simulink model "mdl_VD_dt7dofModel_PPC"  (R2019b)
settings: Solver=ode4  StartTime=0.0  StopTime=50  FixedStep=0.01  RelTol=1e-4  EnableMultiTasking=on
undefined symbols (not defined in the file or in its folder): controller, initial, inputTrajectory, mdlParam, road_properties, vdParam, vehicle
libraries: simulink x9
(part 1 of 2)
settings Model: Creator=cbeal  LastModifiedBy=prasa
settings SolverCC: ZeroCrossAlgorithm=Adaptive
settings DataIOCC: SaveFormat=Array  SaveTime=off  ReturnWorkspaceOutputs=off
settings OptimizationCC: ExpressionDepthLimit=2147483647  LifeSpan=inf
settings DebuggingCC: ReadBeforeWriteMsg=DisableAll  WriteAfterWriteMsg=DisableAll  WriteAfterReadMsg=DisableAll  UnderspecifiedInitializationDetection=Classic  MergeDetectMultiDrivingBlocksExec=none  SolverPrmCheckMsg=warning  MultiTaskDSMMsg=none  FcnCallInpInsideContextMsg=warning  StateNameClashWarn=warning  SFUnexpectedBacktrackingDiag=warning  SFNoUnconditionalDefaultTransitionDiag=warning  SFExecutionAtInitializationDiag=none  ArithmeticOperatorsInVariantConditions=warning
settings HardwareCC: ProdBitPerPointer=32  ProdBitPerSizeT=32  ProdBitPerPtrDiffT=32  ProdLargestAtomicFloat=None  ProdIntDivRoundTo=Undefined  ProdEndianess=Unspecified  ProdWordSize=32  ProdHWDeviceType=32-bit Generic
settings ModelReferenceCC: UpdateModelReferenceTargets=IfOutOfDate  PropagateSignalLabelsOutOfModel=off
settings SFSimCC: SFSimEcho=off  SimUseLocalCustomCode=off  CustomCodeUndefinedFunction=UseInterfaceOnly
settings RTWCC: RTWUseLocalCustomCode=off
settings CodeAppCC: StateflowObjectComments=on
settings GRTTargetCC: TargetLangStandard=C89/C90 (ANSI)
settings ConfigComp: CovMetricSettings=dw  CovHtmlReporting=on  CovSaveCumulativeToWorkspaceVar=on  CovSaveSingleToWorkspaceVar=on  CovExternalEMLEnable=off

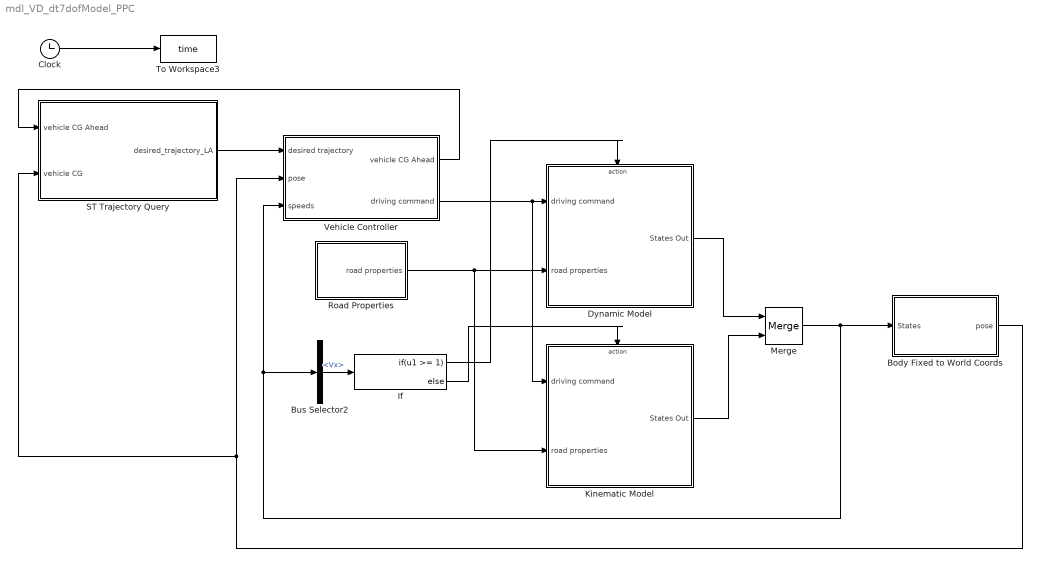
== system mdl_VD_dt7dofModel_PPC ==
  Body Fixed to World Coords : Subsystem
      mask Display: image('$imagefile'); % Use "Edit Image" on toolstrip to change.
  Bus Selector2 : BusSelector  OutputSignals=speeds.Vx
  Clock : Clock
  Dynamic Model : Subsystem
  If : If  IfExpression=u1 >= 1
  Kinematic Model : Subsystem
  Merge : Merge
  Road Properties : Subsystem
  ST Trajectory Query : Subsystem
  To Workspace3 : ToWorkspace  VariableName=time  SampleTime=-1
  Vehicle Controller : Subsystem
  wires:
  Clock/1 -> To Workspace3/1
  Vehicle Controller/2(driving command) -> Kinematic Model/1(driving command), Dynamic Model/1(driving command)
  Road Properties/1(road properties) -> Kinematic Model/2(road properties), Dynamic Model/2(road properties)
  Merge/1 -> Body Fixed to World Coords/1(States), Bus Selector2/1, Vehicle Controller/3(speeds)
  Body Fixed to World Coords/1(pose) -> Vehicle Controller/2(pose), ST Trajectory Query/2(vehicle CG)
  ST Trajectory Query/1(desired_trajectory_LA) -> Vehicle Controller/1(desired trajectory)
  Vehicle Controller/1(vehicle CG Ahead) -> ST Trajectory Query/1(vehicle CG Ahead)
  If/1 -> Dynamic Model/Action
  If/2 -> Kinematic Model/Action
  Bus Selector2/1 -> If/1  "<Vx>"
  Kinematic Model/1(States Out) -> Merge/2
  Dynamic Model/1(States Out) -> Merge/1

== system mdl_VD_dt7dofModel_PPC/Body Fixed to World Coords ==
  States : Inport
  Bus Creator1 : BusCreator  Inputs=3
  Bus Selector4 : BusSelector  OutputSignals=speeds.Vx,speeds.Vy,speeds.r
  Integrator_East : Integrator  InitialCondition=initial.east
  Integrator_North : Integrator  InitialCondition=initial.north
  Integrator_Psi : Integrator  InitialCondition=initial.heading
  Product{4..7} (4 alike) : Product  SaturateOnIntegerOverflow=on  OutDataTypeStr=Inherit: Same as first input
  Sum : Sum  Inputs=+-  SaturateOnIntegerOverflow=on
  Sum1 : Sum  SaturateOnIntegerOverflow=on
  Trigonometric Function2 : Trigonometry
  Trigonometric Function3 : Trigonometry  Operator=cos
  pose : Outport
  wires:
  Bus Creator1/1 -> pose/1
  Product4/1 -> Sum1/1
  Product6/1 -> Sum/2
  Product7/1 -> Sum1/2
  Trigonometric Function2/1 -> Product4/2, Product6/2
  Integrator_Psi/1 -> Bus Creator1/3, Trigonometric Function3/1, Trigonometric Function2/1  "PSI"
  Sum1/1 -> Integrator_North/1
  Sum/1 -> Integrator_East/1
  Trigonometric Function3/1 -> Product5/2, Product7/2
  Integrator_East/1 -> Bus Creator1/1  "East"
  Product5/1 -> Sum/1
  Integrator_North/1 -> Bus Creator1/2  "North"
  Bus Selector4/1 -> Product4/1, Product5/1  "<Vx>"
  Bus Selector4/3 -> Integrator_Psi/1  "<r>"
  Bus Selector4/2 -> Product7/1, Product6/1  "<Vy>"
  States/1 -> Bus Selector4/1

== system mdl_VD_dt7dofModel_PPC/Dynamic Model ==
  driving command : Inport
  road properties : Inport  Port=2
  Action Port : ActionPort  ActionPortLabel=if(u1 >= 1)
  Brush Model : Subsystem
  Normal Force : Subsystem
      mask Display: image('$imagefile'); % Use "Edit Image" on toolstrip to change.
  Slips : Subsystem
      mask Display: image('$imagefile'); % Use "Edit Image" on toolstrip to change.
  Vehicle Body Newtonian Dynamics : Subsystem
      mask Display: image('$imagefile'); % Use "Edit Image" on toolstrip to change.
  States Out : Outport
  wires:
  road properties/1 -> Vehicle Body Newtonian Dynamics/3(Road Geometry), Brush Model/3(Road Friction), Normal Force/2(road properties)
  Normal Force/1(Normal Forces) -> Brush Model/2(Normal Forces)  "Normal Forces"
  Vehicle Body Newtonian Dynamics/1(States_Out) -> States Out/1, Vehicle Body Newtonian Dynamics/4(States_IN), Slips/2(Speeds), Normal Force/1(Accelerations)
  Slips/1(Slips) -> Brush Model/1(Slips)  "Slips"
  driving command/1 -> Vehicle Body Newtonian Dynamics/1(Driving Command), Slips/1(steering angle)
  Brush Model/1(Tire Forces) -> Vehicle Body Newtonian Dynamics/2(Tire Forces)

== system mdl_VD_dt7dofModel_PPC/Kinematic Model ==
  driving command : Inport
  road properties : Inport  Port=2
  Action Port : ActionPort  ActionPortLabel=else
  Constant : Constant  Value=0.015
  Normal Force : Subsystem
      mask Display: image('$imagefile'); % Use "Edit Image" on toolstrip to change.
  Product13 : Product  RndMeth=Zero
  Vehicle Body Newtonian Dynamics : Subsystem
      mask Display: image('$imagefile'); % Use "Edit Image" on toolstrip to change.
  States Out : Outport
  wires:
  road properties/1 -> Vehicle Body Newtonian Dynamics/3(Road Geometry), Normal Force/2(road properties)
  Normal Force/1(Normal Forces) -> Product13/2  "Normal Forces"
  Vehicle Body Newtonian Dynamics/1(States_Out) -> Normal Force/1(Accelerations), States Out/1
  driving command/1 -> Vehicle Body Newtonian Dynamics/1(Driving Command)
  Product13/1 -> Vehicle Body Newtonian Dynamics/2(Rolling Resistance Force)  "Resistive Forces"
  Constant/1 -> Product13/1

== system mdl_VD_dt7dofModel_PPC/Road Properties ==
  Bus Creator1 : BusCreator  Inputs=3
  Bus Creator2 : BusCreator  Inputs=2
  Constant : Constant  Value=road_properties.friction
  Constant1 : Constant  Value=road_properties.grade
  Constant19 : Constant  Value=road_properties.bank_angle
  Constant3 : Constant  Value=0
  road properties : Outport
  wires:
  Constant1/1 -> Bus Creator1/2  "grade"
  Constant19/1 -> Bus Creator1/1  "banking angle"
  Constant3/1 -> Bus Creator1/3  "Curvature"
  Constant/1 -> Bus Creator2/2  "road friction"
  Bus Creator2/1 -> road properties/1  "road properties"
  Bus Creator1/1 -> Bus Creator2/1  "road geometry"

== system mdl_VD_dt7dofModel_PPC/ST Trajectory Query ==
  vehicle CG Ahead : Inport
  vehicle CG : Inport  Port=2
  Constant1 : Constant  Value=mdlParam.max_station
  IsNegative1 : simulink/Logic and Bit Operations/Compare To Zero  relop=<  OutDataTypeStr=boolean
  IsNonNegative1 : simulink/Logic and Bit Operations/Compare To Zero  relop=>=  OutDataTypeStr=boolean
  ST Trajectory Query1 : Subsystem
  ST Trajectory Query2 : Subsystem
  Stop Simulation2 : Stop
  Stop Simulation3 : Stop
  Subtract2 : Sum  Inputs=-+
  Subtract3 : Sum  Inputs=-+
  To Workspace3 : ToWorkspace  VariableName=desired_trajectory  SampleTime=-1
  desired_trajectory_LA : Outport
  wires:
  ST Trajectory Query2/2(desired_trajectory_LA) -> To Workspace3/1, desired_trajectory_LA/1
  vehicle CG/1 -> ST Trajectory Query1/1(vehicle CG(EN))
  vehicle CG Ahead/1 -> ST Trajectory Query2/1(vehicle CG Ahead(EN))
  IsNegative1/1 -> Stop Simulation3/1
  Subtract3/1 -> IsNegative1/1
  Constant1/1 -> Subtract2/1
  IsNonNegative1/1 -> Stop Simulation2/1
  Subtract2/1 -> IsNonNegative1/1
  ST Trajectory Query2/1(vehicle station ahead) -> Subtract3/2
  ST Trajectory Query1/1(vehicle station current) -> Subtract2/2, Subtract3/1

== system mdl_VD_dt7dofModel_PPC/Vehicle Controller ==
  desired trajectory : Inport
  pose : Inport  Port=2
  speeds : Inport  Port=3
  Driver Model : Subsystem
      mask Display: image('$imagefile'); % Use "Edit Image" on toolstrip to change.
  Stabilization : Subsystem
  vehicle CG Ahead : Outport
  driving command : Outport  Port=2
  wires:
  Stabilization/1(driving command) -> driving command/1
  desired trajectory/1 -> Driver Model/1(desired trajectory)
  Driver Model/1(delta) -> Stabilization/1(delta_in)
  Driver Model/2(wheel torque) -> Stabilization/2(wheel torque_in)
  pose/1 -> Driver Model/2(pose)
  Driver Model/3(vehicle CG Ahead) -> vehicle CG Ahead/1
  speeds/1 -> Driver Model/3(speeds)

== system mdl_VD_dt7dofModel_PPC/Dynamic Model/Brush Model ==
  Slips : Inport
  Normal Forces : Inport  Port=2
  Road Friction : Inport  Port=3
  Tire Forces_Brush Model : Subsystem
      mask Display: image('$imagefile'); % Use "Edit Image" on toolstrip to change.
  Tire Forces : Outport
  wires:
  Road Friction/1 -> Tire Forces_Brush Model/3(road friction)
  Tire Forces_Brush Model/1(Tire Forces) -> Tire Forces/1  "Tire Forces"
  Normal Forces/1 -> Tire Forces_Brush Model/2(Normal Forces)
  Slips/1 -> Tire Forces_Brush Model/1(Slips)

== system mdl_VD_dt7dofModel_PPC/Dynamic Model/Normal Force ==
  Accelerations : Inport
  road properties : Inport  Port=2
  Left Front : Sum  Inputs=+--
  Left Rear : Sum  Inputs=++-
  Mux : Mux
  Normal Force Lateral Transfer : Subsystem
      mask Display: image('$imagefile'); % Use "Edit Image" on toolstrip to change.
  Normal Force Longitudinal Transfer : Subsystem
      mask Display: image('$imagefile'); % Use "Edit Image" on toolstrip to change.
  Normal Force Static : Subsystem
  Right Front : Sum  Inputs=+-+
  Right Rear : Sum  Inputs=+++
  To Workspace1 : ToWorkspace  VariableName=Fz  SampleTime=-1
  Normal Forces : Outport
  wires:
  Left Front/1 -> Mux/1
  Right Front/1 -> Mux/2
  Left Rear/1 -> Mux/3
  Right Rear/1 -> Mux/4
  Normal Force Static/4(Static RR) -> Right Rear/1
  Normal Force Static/1(Static FL) -> Left Front/1
  road properties/1 -> Normal Force Static/1(Road Geometry)
  Normal Force Longitudinal Transfer/1(Long Transfer) -> Left Front/2, Right Front/2, Left Rear/2, Right Rear/2
  Accelerations/1 -> Normal Force Lateral Transfer/1(Accelerations), Normal Force Longitudinal Transfer/1(Accelerations)
  Normal Force Lateral Transfer/2(Lateral Transfer Rear) -> Left Rear/3, Right Rear/3
  Normal Force Lateral Transfer/1(Lateral Transfer Front) -> Left Front/3, Right Front/3
  Normal Force Static/3(Static RL) -> Left Rear/1
  Normal Force Static/2(Static FR) -> Right Front/1
  Mux/1 -> To Workspace1/1, Normal Forces/1  "Normal Forces"

== system mdl_VD_dt7dofModel_PPC/Dynamic Model/Slips ==
  steering angle : Inport
  Speeds : Inport  Port=2
  Bus Creator : BusCreator  Inputs=2
  Bus Selector1 : BusSelector  OutputSignals=speeds
  Bus Selector2 : BusSelector  OutputSignals=steering angle
  Slip Angle : Subsystem
      mask Display: image('$imagefile'); % Use "Edit Image" on toolstrip to change.
  To Workspace : ToWorkspace  VariableName=alpha  SampleTime=-1
  To Workspace4 : ToWorkspace  VariableName=kappa  SampleTime=-1
  Wheel Slip Ratio : Subsystem
      mask Display: image('$imagefile'); % Use "Edit Image" on toolstrip to change.
  Slips : Outport
  wires:
  Slip Angle/1(Slip Angles) -> To Workspace/1, Bus Creator/1  "Slip Angles"
  Bus Selector2/1 -> Wheel Slip Ratio/1(delta), Slip Angle/2(delta)  "<steering angle>"
  Wheel Slip Ratio/1(Wheel Slips) -> To Workspace4/1, Bus Creator/2  "Wheel Slips"
  Bus Selector1/1 -> Slip Angle/1(Speeds), Wheel Slip Ratio/2(Speeds)  "<speeds>"
  Bus Creator/1 -> Slips/1
  Speeds/1 -> Bus Selector1/1
  steering angle/1 -> Bus Selector2/1

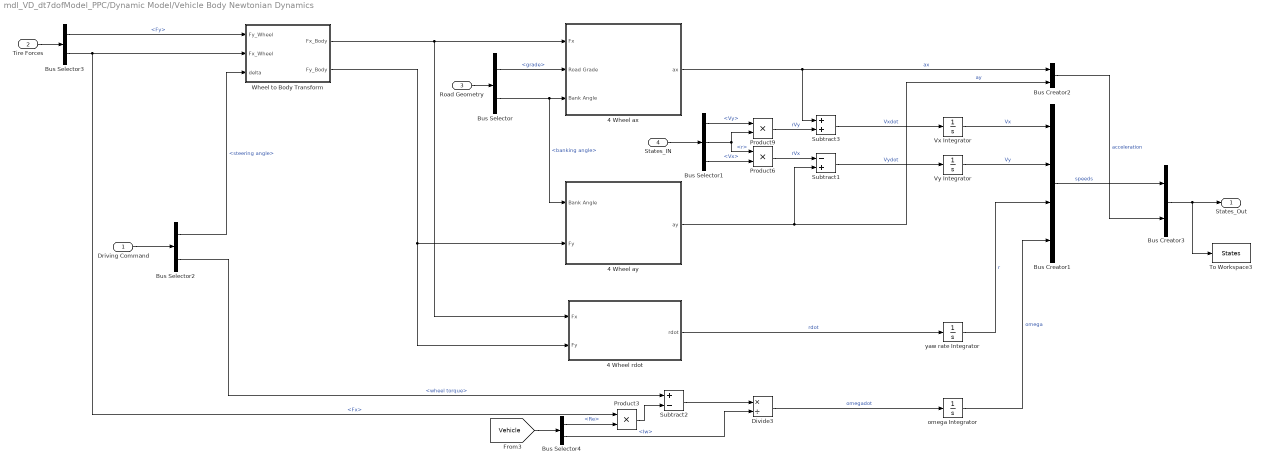
== system mdl_VD_dt7dofModel_PPC/Dynamic Model/Vehicle Body Newtonian Dynamics ==
  Driving Command : Inport
  Tire Forces : Inport  Port=2
  Road Geometry : Inport  Port=3
  States_IN : Inport  Port=4
  4 Wheel ax : Subsystem
  4 Wheel ay : Subsystem
  4 Wheel rdot : Subsystem
  Bus Creator1 : BusCreator  Inputs=4
  Bus Creator2 : BusCreator  Inputs=2
  Bus Creator3 : BusCreator  Inputs=2
  Bus Selector : BusSelector  OutputSignals=road geometry.grade,road geometry.banking angle
  Bus Selector1 : BusSelector  OutputSignals=speeds.Vy,speeds.r,speeds.Vx
  Bus Selector2 : BusSelector  OutputSignals=steering angle,wheel torque
  Bus Selector3 : BusSelector  OutputSignals=Fy,Fx
  Bus Selector4 : BusSelector  OutputSignals=Re,Iw
  Divide3 : Product  Inputs=*/
  Product3 : Product  RndMeth=Zero
  Product6 : Product  RndMeth=Zero
  Product9 : Product  RndMeth=Zero
  Subtract1 : Sum  Inputs=-+
  Subtract2 : Sum  Inputs=+-
  Subtract3 : Sum
  To Workspace3 : ToWorkspace  VariableName=States  SampleTime=-1
  Vx Integrator : Integrator  InitialCondition=initial.longitudinalSpeed
  Vy Integrator : Integrator
  Wheel to Body Transform : Subsystem
  omega Integrator : Integrator  InitialCondition=initial.wheelSpeeds
  yaw rate Integrator : Integrator
  States_Out : Outport
  wires:
  [Vehicle] -> Bus Selector4/1
  Bus Selector4/2 -> Divide3/2  "<Iw>"
  Bus Selector4/1 -> Product3/2  "<Re>"
  Product3/1 -> Subtract2/2
  Subtract2/1 -> Divide3/1
  Divide3/1 -> omega Integrator/1  "omegadot"
  yaw rate Integrator/1 -> Bus Creator1/3  "r"
  Vy Integrator/1 -> Bus Creator1/2  "Vy"
  Vx Integrator/1 -> Bus Creator1/1  "Vx"
  omega Integrator/1 -> Bus Creator1/4  "omega"
  Bus Creator2/1 -> Bus Creator3/2  "acceleration"
  Product6/1 -> Subtract1/1  "rVx"
  Product9/1 -> Subtract3/2  "rVy"
  Subtract3/1 -> Vx Integrator/1  "Vxdot"
  Bus Selector/1 -> 4 Wheel ax/2(Road Grade)  "<grade>"
  Wheel to Body Transform/2(Fy_Body) -> 4 Wheel rdot/2(Fy), 4 Wheel ay/2(Fy)
  Wheel to Body Transform/1(Fx_Body) -> 4 Wheel rdot/1(Fx), 4 Wheel ax/1("Fx ")
  4 Wheel rdot/1(rdot) -> yaw rate Integrator/1  "rdot"
  4 Wheel ay/1(ay) -> Bus Creator2/2, Subtract1/2  "ay"
  4 Wheel ax/1(ax) -> Subtract3/1, Bus Creator2/1  "ax"
  Bus Creator1/1 -> Bus Creator3/1  "speeds"
  Bus Selector/2 -> 4 Wheel ay/1(Bank Angle), 4 Wheel ax/3(Bank Angle)  "<banking angle>"
  Road Geometry/1 -> Bus Selector/1
  Bus Selector2/1 -> Wheel to Body Transform/3(delta)  "<steering angle>"
  States_IN/1 -> Bus Selector1/1
  Bus Selector1/3 -> Product6/2  "<Vx>"
  Bus Selector1/1 -> Product9/1  "<Vy>"
  Bus Selector1/2 -> Product6/1, Product9/2  "<r>"
  Tire Forces/1 -> Bus Selector3/1
  Bus Selector3/2 -> Product3/1, Wheel to Body Transform/2(Fx_Wheel)  "<Fx>"
  Bus Selector3/1 -> Wheel to Body Transform/1(Fy_Wheel)  "<Fy>"
  Driving Command/1 -> Bus Selector2/1
  Bus Selector2/2 -> Subtract2/1  "<wheel torque>"
  Bus Creator3/1 -> To Workspace3/1, States_Out/1
  Subtract1/1 -> Vy Integrator/1  "Vydot"

== system mdl_VD_dt7dofModel_PPC/Kinematic Model/Normal Force ==
  Accelerations : Inport
  road properties : Inport  Port=2
  Left Front : Sum  Inputs=+--
  Left Rear : Sum  Inputs=++-
  Mux : Mux
  Normal Force Lateral Transfer : Subsystem
      mask Display: image('$imagefile'); % Use "Edit Image" on toolstrip to change.
  Normal Force Longitudinal Transfer : Subsystem
      mask Display: image('$imagefile'); % Use "Edit Image" on toolstrip to change.
  Normal Force Static : Subsystem
  Right Front : Sum  Inputs=+-+
  Right Rear : Sum  Inputs=+++
  To Workspace1 : ToWorkspace  VariableName=Fz  SampleTime=-1
  Normal Forces : Outport
  wires:
  Left Front/1 -> Mux/1
  Right Front/1 -> Mux/2
  Left Rear/1 -> Mux/3
  Right Rear/1 -> Mux/4
  Normal Force Static/4(Static RR) -> Right Rear/1
  Normal Force Static/1(Static FL) -> Left Front/1
  road properties/1 -> Normal Force Static/1(Road Geometry)
  Normal Force Longitudinal Transfer/1(Long Transfer) -> Left Front/2, Right Front/2, Left Rear/2, Right Rear/2
  Accelerations/1 -> Normal Force Lateral Transfer/1(Accelerations), Normal Force Longitudinal Transfer/1(Accelerations)
  Normal Force Lateral Transfer/2(Lateral Transfer Rear) -> Left Rear/3, Right Rear/3
  Normal Force Lateral Transfer/1(Lateral Transfer Front) -> Left Front/3, Right Front/3
  Normal Force Static/3(Static RL) -> Left Rear/1
  Normal Force Static/2(Static FR) -> Right Front/1
  Mux/1 -> To Workspace1/1, Normal Forces/1  "Normal Forces"

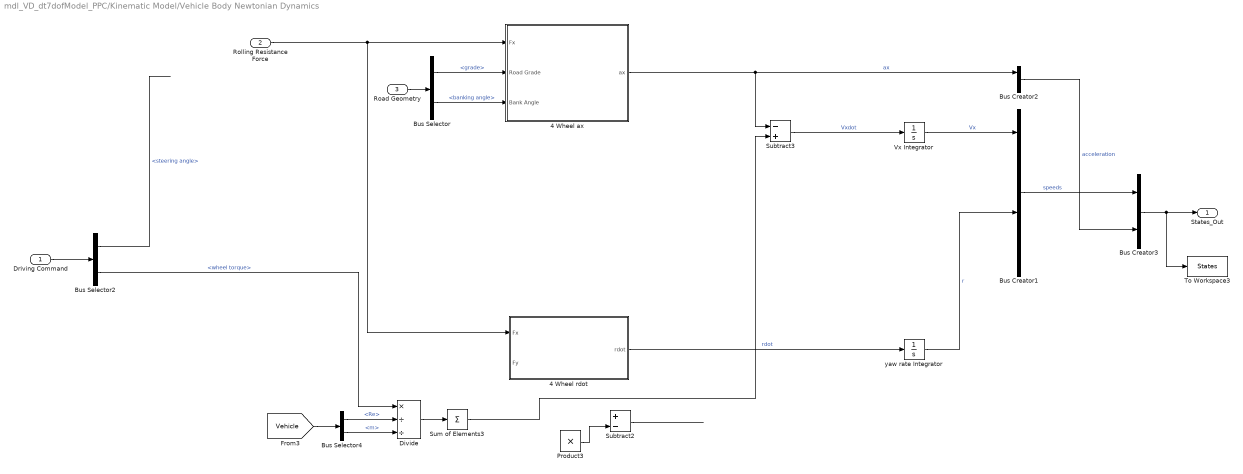
== system mdl_VD_dt7dofModel_PPC/Kinematic Model/Vehicle Body Newtonian Dynamics ==
  Driving Command : Inport
  Rolling Resistance Force : Inport  Port=2
  Road Geometry : Inport  Port=3
  4 Wheel ax : Subsystem
  4 Wheel rdot : Subsystem
  Bus Creator1 : BusCreator  Inputs=4
  Bus Creator2 : BusCreator  Inputs=2
  Bus Creator3 : BusCreator  Inputs=2
  Bus Selector : BusSelector  OutputSignals=road geometry.grade,road geometry.banking angle
  Bus Selector2 : BusSelector  OutputSignals=steering angle,wheel torque
  Bus Selector4 : BusSelector  OutputSignals=Re,m
  Divide : Product  Inputs=*//
  Product3 : Product  RndMeth=Zero
  Subtract2 : Sum  Inputs=+-
  Subtract3 : Sum  Inputs=-+
  Sum of Elements3 : Sum  Inputs=+
  To Workspace3 : ToWorkspace  VariableName=States  SampleTime=-1
  Vx Integrator : Integrator  InitialCondition=initial.longitudinalSpeed
  yaw rate Integrator : Integrator
  States_Out : Outport
  wires:
  [Vehicle] -> Bus Selector4/1
  Bus Selector4/1 -> Divide/2  "<Re>"
  Product3/1 -> Subtract2/2
  Subtract2/1 -> ?
  ? -> ?  "omegadot"
  yaw rate Integrator/1 -> Bus Creator1/3  "r"
  ? -> Bus Creator1/2  "Vy"
  Vx Integrator/1 -> Bus Creator1/1  "Vx"
  ? -> Bus Creator1/4  "omega"
  Bus Creator2/1 -> Bus Creator3/2  "acceleration"
  Subtract3/1 -> Vx Integrator/1  "Vxdot"
  Bus Selector/1 -> 4 Wheel ax/2(Road Grade)  "<grade>"
  ? -> 4 Wheel rdot/2(Fy)
  Rolling Resistance Force/1 -> 4 Wheel rdot/1(Fx), 4 Wheel ax/1("Fx ")
  4 Wheel rdot/1(rdot) -> yaw rate Integrator/1  "rdot"
  ? -> Bus Creator2/2  "ay"
  4 Wheel ax/1(ax) -> Subtract3/1, Bus Creator2/1  "ax"
  Bus Creator1/1 -> Bus Creator3/1  "speeds"
  Bus Selector/2 -> 4 Wheel ax/3(Bank Angle)  "<banking angle>"
  Road Geometry/1 -> Bus Selector/1
  Bus Selector2/1 -> ?  "<steering angle>"
  Driving Command/1 -> Bus Selector2/1
  Bus Selector2/2 -> Divide/1  "<wheel torque>"
  Bus Creator3/1 -> To Workspace3/1, States_Out/1
  Bus Selector4/2 -> Divide/3  "<m>"
  Divide/1 -> Sum of Elements3/1
  Sum of Elements3/1 -> Subtract3/2

== system mdl_VD_dt7dofModel_PPC/ST Trajectory Query/ST Trajectory Query1 ==
  vehicle CG(EN) : Inport
  Bus Creator1 : BusCreator  Inputs=2
  Bus Creator3 : BusCreator  Inputs=16
  Bus Creator8 : BusCreator  Inputs=2
  Bus Selector1 : BusSelector  OutputSignals=East,North
  Demux2 : Demux  Outputs=16
  Selector1 : Selector  NumberOfDimensions=2  InputPortWidth=3  IndexOptions=Starting index (dialog),Starting index (dialog)  Indices=[1],1  OutputSizes=1,16
  To Workspace1 : ToWorkspace  VariableName=vehicle_station  SampleTime=-1
      settings: Save2DSignal=2-D array (concatenate along first dimension)
  To Workspace2 : ToWorkspace  VariableName=pose  SampleTime=-1
  Trajectory Query Block : M-S-Function  FunctionName=sfcn_VD_snapPointOntoNearestTrajectory  Parameters=fieldsTrajectory, mdlParam.searchDistance, mdlParam.trajectorySize
      settings: AttributesFormatString=%<BlockType>
  Vehicle Parameters : Subsystem  mask{vehicleName='C5 Vette', m=1600, Izz=2500, Iw=1.2, Re=0.32, a=1.3, b=1.3, d=1.5, h_cg=0.42, Ca=[95000; 95000; 110000; 110000], Cx=[65000,65000,65000,65000]}
      mask prompts: vehicleName "Name of Vehicle"; m "Mass"; Izz "Yaw Moment of Inertia"; Iw "Wheel Moment of Inertia"; Re "Wheel Effective Radius"; a "CG-Front Axle Distance"; b "CG-Rear Axle Distance"; d "Track Width"; h_cg "CG height"; Ca "Cornering Stiffnesses (x4)"; Cx "Longitudinal Stiffnesses (x4)"
      mask Display: port_label('output',1,vehicleName)
  vehicle_trajectory : Constant  Value=inputTrajectory
  vehicle station current : Outport
  tag scope: Vehicle=global
  wires:
  Trajectory Query Block/1 -> Selector1/1
  vehicle CG(EN)/1 -> Bus Creator8/1, Bus Selector1/1
  vehicle_trajectory/1 -> Trajectory Query Block/1
  Bus Creator1/1 -> Trajectory Query Block/2
  Bus Selector1/2 -> Bus Creator1/2  "<North>"
  Bus Selector1/1 -> Bus Creator1/1  "<East>"
  Demux2/16 -> Bus Creator3/16  "Des Heading"
  Vehicle Parameters/1(Vehicle) -> [Vehicle]
  Demux2/13 -> Bus Creator3/13, vehicle station current/1, To Workspace1/1  "Total Station"
  Demux2/9 -> Bus Creator3/9  "Des CG East"
  Demux2/14 -> Bus Creator3/14  "AIMSUN Time"
  Demux2/7 -> Bus Creator3/7  "Lane Number"
  Bus Creator3/1 -> Vehicle Parameters/1(In1)
  Demux2/12 -> Bus Creator3/12  "Des Velocity"
  Demux2/6 -> Bus Creator3/6  "Junction ID"
  Selector1/1 -> Demux2/1
  Demux2/1 -> Bus Creator3/1  "Vehicle ID"
  Demux2/3 -> Bus Creator3/3  "L"
  Demux2/2 -> Bus Creator3/2  "Vehicle Type"
  Demux2/5 -> Bus Creator3/5  "Section ID"
  Demux2/10 -> Bus Creator3/10  "Des CG North"
  Demux2/4 -> Bus Creator3/4  "d"
  Demux2/8 -> Bus Creator3/8  "Lane Change Flag"
  Bus Creator8/1 -> To Workspace2/1
  Demux2/11 -> Bus Creator3/11, Bus Creator8/2  "Des CG Up"
  Demux2/15 -> Bus Creator3/15  "SysGen Time"

== system mdl_VD_dt7dofModel_PPC/ST Trajectory Query/ST Trajectory Query2 ==
  vehicle CG Ahead(EN) : Inport
  Bus Creator1 : BusCreator  Inputs=8
  Bus Creator2 : BusCreator  Inputs=5
  Bus Creator4 : BusCreator  Inputs=3
  Demux1 : Demux  Outputs=3
  Demux2 : Demux  Outputs=16
  Memory : Memory
  Mux1 : Mux  Inputs=2
  Selector1 : Selector  NumberOfDimensions=2  InputPortWidth=3  IndexOptions=Starting index (dialog),Starting index (dialog)  Indices=[1],1  OutputSizes=1,16
  Terminator : Terminator
  Terminator1 : Terminator
  Terminator2 : Terminator
  Trajectory Query Block : M-S-Function  FunctionName=sfcn_VD_snapPointOntoNearestTrajectory1  Parameters=fieldsTrajectory, mdlParam.searchDistance, mdlParam.trajectorySize
      settings: AttributesFormatString=%<BlockType>
  vehicle_trajectory : Constant  Value=inputTrajectory
  vehicle station ahead : Outport
  desired_trajectory_LA : Outport  Port=2
  wires:
  vehicle CG Ahead(EN)/1 -> Demux1/1
  Demux1/2 -> Mux1/2  "North"
  vehicle_trajectory/1 -> Trajectory Query Block/1
  Trajectory Query Block/1 -> Selector1/1
  Mux1/1 -> Trajectory Query Block/2
  Demux2/3 -> Bus Creator1/3  "L"
  Demux2/2 -> Bus Creator1/2  "Vehicle Type"
  Demux2/8 -> Bus Creator1/8  "Lane Change Flag"
  Demux2/4 -> Bus Creator1/4  "d"
  Demux2/14 -> Bus Creator4/2  "AIMSUN Time"
  Demux2/5 -> Bus Creator1/5  "Section ID"
  Demux2/10 -> Bus Creator2/2  "Des CG North"
  Demux2/13 -> vehicle station ahead/1, Bus Creator4/1  "Total Station"
  Demux2/16 -> Bus Creator2/5  "Des Heading"
  Demux2/11 -> Memory/1  "Des CG Up"
  Selector1/1 -> Demux2/1
  Demux2/1 -> Bus Creator1/1  "Vehicle ID"
  Demux2/6 -> Bus Creator1/6  "Junction ID"
  Demux2/15 -> Bus Creator4/3  "SysGen Time"
  Demux2/7 -> Bus Creator1/7  "Lane Number"
  Demux2/9 -> Bus Creator2/1  "Des CG East"
  Bus Creator1/1 -> Terminator/1
  Demux2/12 -> Bus Creator2/4  "Des Velocity"
  Bus Creator2/1 -> desired_trajectory_LA/1
  Bus Creator4/1 -> Terminator1/1
  Memory/1 -> Bus Creator2/3  "Des CG Up"
  Demux1/1 -> Mux1/1  "East"
  Demux1/3 -> Terminator2/1

== system mdl_VD_dt7dofModel_PPC/Vehicle Controller/Driver Model ==
  desired trajectory : Inport
  pose : Inport  Port=2
  speeds : Inport  Port=3
  Steering Control : Subsystem
      mask Display: image('$imagefile'); % Use "Edit Image" on toolstrip to change.
  Velocity Control : Subsystem
  delta : Outport
  wheel torque : Outport  Port=2
  vehicle CG Ahead : Outport  Port=3
  wires:
  desired trajectory/1 -> Velocity Control/1(desired velocity), Steering Control/2(desired trajectory)
  pose/1 -> Steering Control/1(pose)
  Steering Control/1(steering angle) -> delta/1
  Velocity Control/1(wheel torque) -> wheel torque/1
  Steering Control/2(vehicle CG Ahead) -> vehicle CG Ahead/1
  speeds/1 -> Velocity Control/2(speeds)

== system mdl_VD_dt7dofModel_PPC/Vehicle Controller/Stabilization ==
  delta_in : Inport
  wheel torque_in : Inport  Port=2
  Bus Creator1 : BusCreator  Inputs=2
  Gain : Gain
  Gain1 : Gain
  To Workspace12 : ToWorkspace  VariableName=wheel_torque  SampleTime=-1
  To Workspace3 : ToWorkspace  VariableName=delta  SampleTime=-1
  steering angle limitation : Saturate  UpperLimit=30*pi/180  LowerLimit=-30*pi/180
  torque limitation : Saturate  UpperLimit=200  LowerLimit=-400
  driving command : Outport
  wires:
  wheel torque_in/1 -> Gain/1
  delta_in/1 -> Gain1/1
  Gain/1 -> torque limitation/1
  Gain1/1 -> steering angle limitation/1
  steering angle limitation/1 -> To Workspace3/1, Bus Creator1/1  "steering angle"
  Bus Creator1/1 -> driving command/1
  torque limitation/1 -> To Workspace12/1, Bus Creator1/2  "wheel torque"

== system mdl_VD_dt7dofModel_PPC/Dynamic Model/Brush Model/Tire Forces_Brush Model ==
  note: ISO Coordinate System
  note: [1] J. Svendenius, “Tire Modeling and Friction Estimation,” Control , p. 194, 2007. chapter2.4 and chapter4
      | [2] M. Kissai et al. , “A new linear tire model with varying parameters To cite this version : HAL Id : hal-01690792 A New Linear Tire Model With Varying Parameters,” 2018.
  Slips : Inport
  Normal Forces : Inport  Port=2
  road friction : Inport  Port=3
  Bus Selector2 : BusSelector  OutputSignals=road friction
  Constant3 : Constant
  Switch1 : Switch  Threshold=1  ZeroCross=off
  Wheel Forces : Subsystem
  tire slip : Subsystem
  Tire Forces : Outport
  wires:
  tire slip/1(sigma_x) -> Wheel Forces/3(sigma_x)
  Normal Forces/1 -> tire slip/2(normal force), Wheel Forces/2(normal force)
  tire slip/4(Psi_Tire) -> Switch1/3, Switch1/2
  tire slip/2(sigma_y) -> Wheel Forces/4(sigma_y)
  tire slip/3(sigma) -> Wheel Forces/5(sigma)
  Bus Selector2/1 -> Wheel Forces/1(sliding friction), tire slip/1(peak friction)  "<road friction>"
  Wheel Forces/1(Tire Forces) -> Tire Forces/1
  Constant3/1 -> Switch1/1  "Pure Sliding"
  Switch1/1 -> Wheel Forces/6(Psi_Tire)
  Slips/1 -> tire slip/3(Slips)
  road friction/1 -> Bus Selector2/1

== system mdl_VD_dt7dofModel_PPC/Dynamic Model/Normal Force/Normal Force Lateral Transfer ==
  Accelerations : Inport
  Bus Selector1 : BusSelector  OutputSignals=acceleration.ay
  Bus Selector4 : BusSelector  OutputSignals=b,L,a
  Bus Selector6 : BusSelector  OutputSignals=m,h_cg,d
  Compare To Constant : simulink/Logic and Bit Operations/Compare To Constant  relop===  const=1  OutDataTypeStr=boolean
  Constant : Constant  Value=vdParam.lateralTransfer
  Delay : Delay  DelayLength=1  InitialCondition=0
  Divide3 : Product  Inputs=*/
  Divide4 : Product  Inputs=/*
  Product{1..2,4..6} (5 alike) : Product  RndMeth=Zero
  Product3 : Product  Inputs=*/  RndMeth=Zero
  Lateral Transfer Front : Outport
  Lateral Transfer Rear : Outport  Port=2
  wires:
  Divide3/1 -> Product2/2
  Bus Selector4/2 -> Divide3/2, Divide4/1  "<L>"
  Bus Selector4/1 -> Divide3/1  "<b>"
  Product6/1 -> Product5/1
  Product2/1 -> Lateral Transfer Front/1
  Product5/1 -> Product2/1, Product1/2
  Bus Selector6/2 -> Product3/1  "<h_cg>"
  Product1/1 -> Lateral Transfer Rear/1
  Bus Selector6/1 -> Product4/2  "<m>"
  Accelerations/1 -> Bus Selector1/1
  Divide4/1 -> Product1/1
  Bus Selector1/1 -> Delay/1  "<ay>"
  Bus Selector6/3 -> Product3/2  "<d>"
  [Vehicle] -> Bus Selector4/1
  [Vehicle] -> Bus Selector6/1
  Bus Selector4/3 -> Divide4/2  "<a>"
  Product4/1 -> Product6/2
  Product3/1 -> Product5/2
  Compare To Constant/1 -> Product6/1
  Constant/1 -> Compare To Constant/1
  Delay/1 -> Product4/1

== system mdl_VD_dt7dofModel_PPC/Dynamic Model/Normal Force/Normal Force Longitudinal Transfer ==
  Accelerations : Inport
  Bus Selector2 : BusSelector  OutputSignals=m,L,h_cg
  Bus Selector3 : BusSelector  OutputSignals=acceleration.ax
  Compare To Constant : simulink/Logic and Bit Operations/Compare To Constant  relop===  const=1  OutDataTypeStr=boolean
  Constant : Constant  Value=vdParam.longitudinalTransfer
  Delay : Delay  DelayLength=1  InitialCondition=0
  Divide1 : Product  Inputs=/*
  Gain3 : Gain  Gain=2
  Product1 : Product  RndMeth=Zero
  Product2 : Product  RndMeth=Zero
  Product3 : Product  RndMeth=Zero
  Long Transfer : Outport
  wires:
  Bus Selector2/2 -> Gain3/1  "<L>"
  Product3/1 -> Product1/1
  Bus Selector2/3 -> Divide1/2  "<h_cg>"
  Divide1/1 -> Product1/2
  [Vehicle] -> Bus Selector2/1
  Bus Selector2/1 -> Product2/2  "<m>"
  Bus Selector3/1 -> Delay/1  "<ax>"
  Product2/1 -> Product3/2
  Product1/1 -> Long Transfer/1
  Gain3/1 -> Divide1/1
  Accelerations/1 -> Bus Selector3/1
  Compare To Constant/1 -> Product3/1
  Constant/1 -> Compare To Constant/1
  Delay/1 -> Product2/1

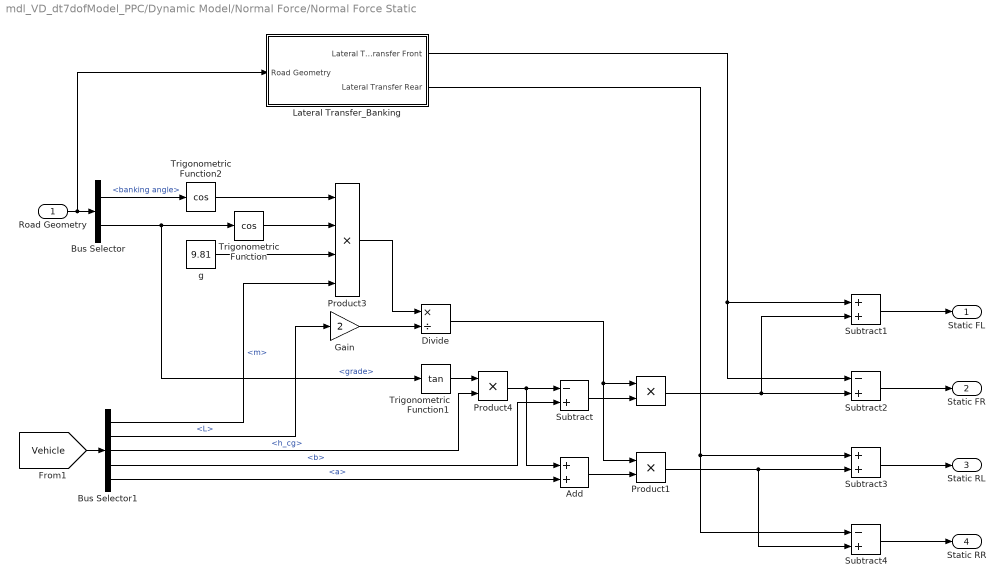
== system mdl_VD_dt7dofModel_PPC/Dynamic Model/Normal Force/Normal Force Static ==
  Road Geometry : Inport
  " " : Product  RndMeth=Zero
  Add : Sum
  Bus Selector : BusSelector  OutputSignals=road geometry.banking angle,road geometry.grade
  Bus Selector1 : BusSelector  OutputSignals=m,L,h_cg,b,a
  Divide : Product  Inputs=*/
  Gain : Gain  Gain=2
  Lateral Transfer_Banking : Subsystem
  Product1 : Product  RndMeth=Zero
  Product3 : Product  Inputs=4  RndMeth=Zero
  Product4 : Product  RndMeth=Zero
  Subtract : Sum  Inputs=-+
  Subtract1 : Sum
  Subtract2 : Sum  Inputs=-+
  Subtract3 : Sum
  Subtract4 : Sum  Inputs=-+
  Trigonometric Function : Trigonometry  Operator=cos
  Trigonometric Function1 : Trigonometry  Operator=tan
  Trigonometric Function2 : Trigonometry  Operator=cos
  g : Constant  Value=9.81
  Static FL : Outport
  Static FR : Outport  Port=2
  Static RL : Outport  Port=3
  Static RR : Outport  Port=4
  wires:
  Product4/1 -> Add/1, Subtract/1
  Add/1 -> Product1/2
  g/1 -> Product3/3
  [Vehicle] -> Bus Selector1/1
  Bus Selector1/4 -> Subtract/2  "<b>"
  Product3/1 -> Divide/1
  Bus Selector1/1 -> Product3/4  "<m>"
  Trigonometric Function/1 -> Product3/2
  Bus Selector1/5 -> Add/2  "<a>"
  Bus Selector1/3 -> Product4/2  "<h_cg>"
  Trigonometric Function1/1 -> Product4/1
  Divide/1 -> Product1/1, " "/1
  Bus Selector/2 -> Trigonometric Function1/1, Trigonometric Function/1  "<grade>"
  Bus Selector1/2 -> Gain/1  "<L>"
  Subtract/1 -> " "/2
  Gain/1 -> Divide/2
  Road Geometry/1 -> Lateral Transfer_Banking/1(Road Geometry), Bus Selector/1
  Product1/1 -> Subtract4/2, Subtract3/2
  " "/1 -> Subtract2/2, Subtract1/2
  Trigonometric Function2/1 -> Product3/1
  Bus Selector/1 -> Trigonometric Function2/1  "<banking angle>"
  Subtract4/1 -> Static RR/1
  Subtract3/1 -> Static RL/1
  Subtract2/1 -> Static FR/1
  Subtract1/1 -> Static FL/1
  Lateral Transfer_Banking/2(Lateral Transfer Rear) -> Subtract3/1, Subtract4/1
  Lateral Transfer_Banking/1(Lateral Transfer Front) -> Subtract2/1, Subtract1/1

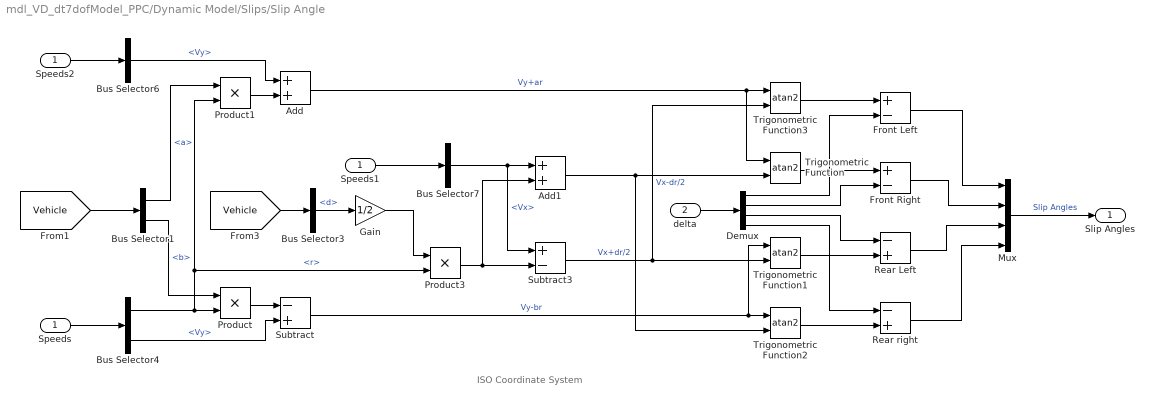
== system mdl_VD_dt7dofModel_PPC/Dynamic Model/Slips/Slip Angle ==
  note: ISO Coordinate System
  Speeds : Inport
  delta : Inport  Port=2
  Add : Sum
  Add1 : Sum
  Bus Selector1 : BusSelector  OutputSignals=a,b
  Bus Selector3 : BusSelector  OutputSignals=d
  Bus Selector4 : BusSelector  OutputSignals=r,Vy
  Bus Selector6 : BusSelector  OutputSignals=Vy
  Bus Selector7 : BusSelector  OutputSignals=Vx
  Demux : Demux
  Front Left : Sum  Inputs=+-
  Front Right : Sum  Inputs=+-
  Gain : Gain  Gain=1/2
  Mux : Mux
  Product : Product  RndMeth=Zero
  Product1 : Product  RndMeth=Zero
  Product3 : Product  RndMeth=Zero
  Rear Left : Sum  Inputs=-+
  Rear right : Sum  Inputs=-+
  Speeds1 : InportShadow
  Speeds2 : InportShadow
  Subtract : Sum  Inputs=-+
  Subtract3 : Sum  Inputs=+-
  Trigonometric Function{,1..3} (4 alike) : Trigonometry  Operator=atan2
  Slip Angles : Outport
  wires:
  Speeds1/1 -> Bus Selector7/1
  Bus Selector4/1 -> Product1/2, Product3/2, Product/2  "<r>"
  Demux/1 -> Front Left/2
  Subtract/1 -> Trigonometric Function2/1, Trigonometric Function1/1  "Vy-br"
  Add1/1 -> Trigonometric Function/2, Trigonometric Function2/2  "Vx+dr/2"
  Product3/1 -> Add1/2, Subtract3/2
  Demux/2 -> Front Right/2
  Trigonometric Function1/1 -> Rear Left/2
  Subtract3/1 -> Trigonometric Function3/2, Trigonometric Function1/2  "Vx-dr/2"
  Trigonometric Function/1 -> Front Right/1
  Gain/1 -> Product3/1
  delta/1 -> Demux/1
  Rear Left/1 -> Mux/3
  Rear right/1 -> Mux/4
  Bus Selector3/1 -> Gain/1  "<d>"
  Demux/4 -> Rear right/1
  Demux/3 -> Rear Left/1
  Add/1 -> Trigonometric Function/1, Trigonometric Function3/1  "Vy+ar"
  [Vehicle] -> Bus Selector1/1
  Product/1 -> Subtract/1
  Mux/1 -> Slip Angles/1  "Slip Angles"
  Trigonometric Function2/1 -> Rear right/2
  Bus Selector1/2 -> Product/1  "<b>"
  Front Right/1 -> Mux/2
  Front Left/1 -> Mux/1
  [Vehicle] -> Bus Selector3/1
  Bus Selector1/1 -> Product1/1  "<a>"
  Trigonometric Function3/1 -> Front Left/1
  Product1/1 -> Add/2
  Bus Selector7/1 -> Subtract3/1, Add1/1  "<Vx>"
  Speeds2/1 -> Bus Selector6/1
  Bus Selector4/2 -> Subtract/2  "<Vy>"
  Bus Selector6/1 -> Add/1  "<Vy>"
  Speeds/1 -> Bus Selector4/1

== system mdl_VD_dt7dofModel_PPC/Dynamic Model/Slips/Wheel Slip Ratio ==
  delta : Inport
  Speeds : Inport  Port=2
  Wheel Slip : Subsystem
  vehicle2tire : Subsystem
  Wheel Slips : Outport
  wires:
  Speeds/1 -> vehicle2tire/2(Speeds), Wheel Slip/2(Speeds)  "Vx,Vy,r,omega"
  delta/1 -> vehicle2tire/1(delta)
  vehicle2tire/1(Vx_tire) -> Wheel Slip/1(Vx_tire)
  Wheel Slip/1(Wheel Slips) -> Wheel Slips/1

== system mdl_VD_dt7dofModel_PPC/Dynamic Model/Vehicle Body Newtonian Dynamics/4 Wheel ax ==
  "Fx " : Inport
  Road Grade : Inport  Port=2
  Bank Angle : Inport  Port=3
  Add2 : Sum  Inputs=-+
  Bus Selector6 : BusSelector  OutputSignals=m
  Bus Selector7 : BusSelector  OutputSignals=m
  Divide2 : Product  Inputs=/*
  Product10 : Product  Inputs=4  RndMeth=Zero
  Sum of Elements3 : Sum  Inputs=+
  cos : Trigonometry  Operator=cos
  g : Constant  Value=9.81
  sin : Trigonometry
  ax : Outport
  wires:
  [Vehicle] -> Bus Selector6/1
  [Vehicle] -> Bus Selector7/1
  Add2/1 -> Divide2/2
  Bus Selector7/1 -> Divide2/1  "<m>"
  Divide2/1 -> ax/1
  Product10/1 -> Add2/1
  Sum of Elements3/1 -> Add2/2
  Bus Selector6/1 -> Product10/4  "<m>"
  g/1 -> Product10/3
  sin/1 -> Product10/1
  cos/1 -> Product10/2
  Bank Angle/1 -> cos/1
  Road Grade/1 -> sin/1
  "Fx "/1 -> Sum of Elements3/1

== system mdl_VD_dt7dofModel_PPC/Dynamic Model/Vehicle Body Newtonian Dynamics/4 Wheel ay ==
  Bank Angle : Inport
  Fy : Inport  Port=2
  Add : Sum
  Bus Selector2 : BusSelector  OutputSignals=m
  Bus Selector5 : BusSelector  OutputSignals=m
  Divide1 : Product  Inputs=*/
  Product4 : Product  Inputs=3  RndMeth=Zero
  Sum of Elements : Sum  Inputs=+
  g : Constant  Value=9.81
  sin : Trigonometry
  ay : Outport
  wires:
  [Vehicle] -> Bus Selector2/1
  Fy/1 -> Sum of Elements/1
  Product4/1 -> Add/2
  Add/1 -> Divide1/1
  Bus Selector2/1 -> Divide1/2  "<m>"
  Divide1/1 -> ay/1
  [Vehicle] -> Bus Selector5/1
  g/1 -> Product4/2
  Bus Selector5/1 -> Product4/1  "<m>"
  sin/1 -> Product4/3
  Bank Angle/1 -> sin/1
  Sum of Elements/1 -> Add/1

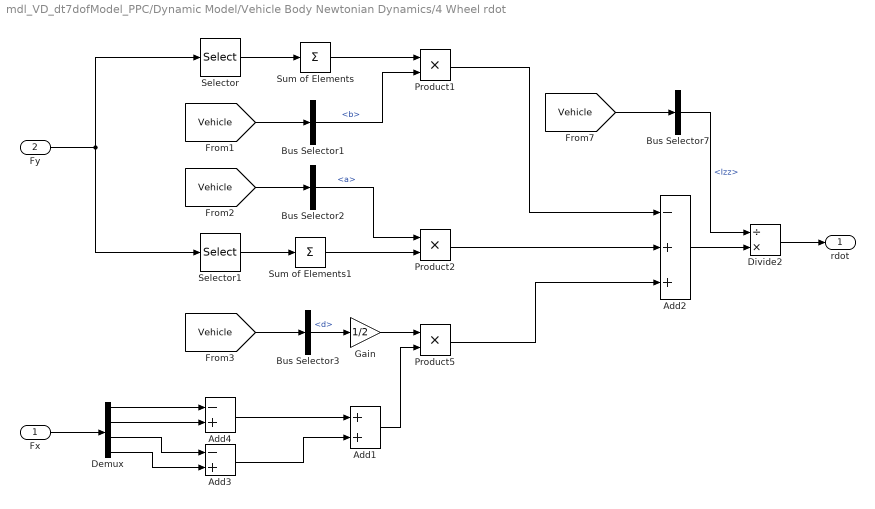
== system mdl_VD_dt7dofModel_PPC/Dynamic Model/Vehicle Body Newtonian Dynamics/4 Wheel rdot ==
  Fx : Inport
  Fy : Inport  Port=2
  Add1 : Sum
  Add2 : Sum  Inputs=-++
  Add3 : Sum  Inputs=-+
  Add4 : Sum  Inputs=-+
  Bus Selector1 : BusSelector  OutputSignals=b
  Bus Selector2 : BusSelector  OutputSignals=a
  Bus Selector3 : BusSelector  OutputSignals=d
  Bus Selector7 : BusSelector  OutputSignals=Izz
  Demux : Demux
  Divide2 : Product  Inputs=/*
  Gain : Gain  Gain=1/2
  Product1 : Product  RndMeth=Zero
  Product2 : Product  RndMeth=Zero
  Product5 : Product  RndMeth=Zero
  Selector : Selector  InputPortWidth=4  IndexOptions=Index vector (dialog)  Indices=[3 4]  OutputSizes=1
  Selector1 : Selector  InputPortWidth=4  IndexOptions=Index vector (dialog)  Indices=[1 2]  OutputSizes=1
  Sum of Elements : Sum  Inputs=+
  Sum of Elements1 : Sum  Inputs=+
  rdot : Outport
  wires:
  Fy/1 -> Selector/1, Selector1/1
  Divide2/1 -> rdot/1
  Bus Selector7/1 -> Divide2/1  "<Izz>"
  Add2/1 -> Divide2/2
  [Vehicle] -> Bus Selector7/1
  [Vehicle] -> Bus Selector1/1
  Selector/1 -> Sum of Elements/1
  Selector1/1 -> Sum of Elements1/1
  Sum of Elements/1 -> Product1/1
  Bus Selector1/1 -> Product1/2  "<b>"
  Product1/1 -> Add2/1
  Fx/1 -> Demux/1
  [Vehicle] -> Bus Selector2/1
  Product2/1 -> Add2/2
  Bus Selector2/1 -> Product2/1  "<a>"
  Sum of Elements1/1 -> Product2/2
  Demux/3 -> Add3/1
  Demux/4 -> Add3/2
  Demux/1 -> Add4/1
  Demux/2 -> Add4/2
  Add4/1 -> Add1/1
  [Vehicle] -> Bus Selector3/1
  Add1/1 -> Product5/2
  Bus Selector3/1 -> Gain/1  "<d>"
  Gain/1 -> Product5/1
  Product5/1 -> Add2/3
  Add3/1 -> Add1/2

== system mdl_VD_dt7dofModel_PPC/Dynamic Model/Vehicle Body Newtonian Dynamics/Wheel to Body Transform ==
  note: ISO Coordinate Transform
  Fy_Wheel : Inport
  Fx_Wheel : Inport  Port=2
  delta : Inport  Port=3
  Add : Sum
  Cos1 : Trigonometry
  Cos2 : Trigonometry  Operator=cos
  Cos8 : Trigonometry  Operator=cos
  Cos9 : Trigonometry
  Fx_Wheel1 : InportShadow  Port=2
  Fy_Wheel1 : InportShadow
  Product{4..7} (4 alike) : Product
  Subtract : Sum  Inputs=+-
  Fx_Body : Outport
  Fy_Body : Outport  Port=2
  wires:
  Subtract/1 -> Fx_Body/1
  delta/1 -> Cos8/1, Cos9/1, Cos2/1, Cos1/1
  Cos8/1 -> Product4/1
  Cos9/1 -> Product5/1
  Cos1/1 -> Product6/1
  Cos2/1 -> Product7/1
  Fx_Wheel1/1 -> Product6/2
  Fy_Wheel1/1 -> Product7/2
  Fy_Wheel/1 -> Product5/2
  Fx_Wheel/1 -> Product4/2
  Product4/1 -> Subtract/1
  Product5/1 -> Subtract/2
  Product6/1 -> Add/1
  Product7/1 -> Add/2
  Add/1 -> Fy_Body/1

== system mdl_VD_dt7dofModel_PPC/Kinematic Model/Normal Force/Normal Force Lateral Transfer ==
  Accelerations : Inport
  Bus Selector1 : BusSelector  OutputSignals=acceleration.ay
  Bus Selector4 : BusSelector  OutputSignals=b,L,a
  Bus Selector6 : BusSelector  OutputSignals=m,h_cg,d
  Compare To Constant : simulink/Logic and Bit Operations/Compare To Constant  relop===  const=1  OutDataTypeStr=boolean
  Constant : Constant  Value=vdParam.lateralTransfer
  Delay : Delay  DelayLength=1  InitialCondition=0
  Divide3 : Product  Inputs=*/
  Divide4 : Product  Inputs=/*
  Product{1..2,4..6} (5 alike) : Product  RndMeth=Zero
  Product3 : Product  Inputs=*/  RndMeth=Zero
  Lateral Transfer Front : Outport
  Lateral Transfer Rear : Outport  Port=2
  wires:
  Divide3/1 -> Product2/2
  Bus Selector4/2 -> Divide3/2, Divide4/1  "<L>"
  Bus Selector4/1 -> Divide3/1  "<b>"
  Product6/1 -> Product5/1
  Product2/1 -> Lateral Transfer Front/1
  Product5/1 -> Product2/1, Product1/2
  Bus Selector6/2 -> Product3/1  "<h_cg>"
  Product1/1 -> Lateral Transfer Rear/1
  Bus Selector6/1 -> Product4/2  "<m>"
  Accelerations/1 -> Bus Selector1/1
  Divide4/1 -> Product1/1
  Bus Selector1/1 -> Delay/1  "<ay>"
  Bus Selector6/3 -> Product3/2  "<d>"
  [Vehicle] -> Bus Selector4/1
  [Vehicle] -> Bus Selector6/1
  Bus Selector4/3 -> Divide4/2  "<a>"
  Product4/1 -> Product6/2
  Product3/1 -> Product5/2
  Compare To Constant/1 -> Product6/1
  Constant/1 -> Compare To Constant/1
  Delay/1 -> Product4/1

== system mdl_VD_dt7dofModel_PPC/Kinematic Model/Normal Force/Normal Force Longitudinal Transfer ==
  Accelerations : Inport
  Bus Selector2 : BusSelector  OutputSignals=m,L,h_cg
  Bus Selector3 : BusSelector  OutputSignals=acceleration.ax
  Compare To Constant : simulink/Logic and Bit Operations/Compare To Constant  relop===  const=1  OutDataTypeStr=boolean
  Constant : Constant  Value=vdParam.longitudinalTransfer
  Delay : Delay  DelayLength=1  InitialCondition=0
  Divide1 : Product  Inputs=/*
  Gain3 : Gain  Gain=2
  Product1 : Product  RndMeth=Zero
  Product2 : Product  RndMeth=Zero
  Product3 : Product  RndMeth=Zero
  Long Transfer : Outport
  wires:
  Bus Selector2/2 -> Gain3/1  "<L>"
  Product3/1 -> Product1/1
  Bus Selector2/3 -> Divide1/2  "<h_cg>"
  Divide1/1 -> Product1/2
  [Vehicle] -> Bus Selector2/1
  Bus Selector2/1 -> Product2/2  "<m>"
  Bus Selector3/1 -> Delay/1  "<ax>"
  Product2/1 -> Product3/2
  Product1/1 -> Long Transfer/1
  Gain3/1 -> Divide1/1
  Accelerations/1 -> Bus Selector3/1
  Compare To Constant/1 -> Product3/1
  Constant/1 -> Compare To Constant/1
  Delay/1 -> Product2/1

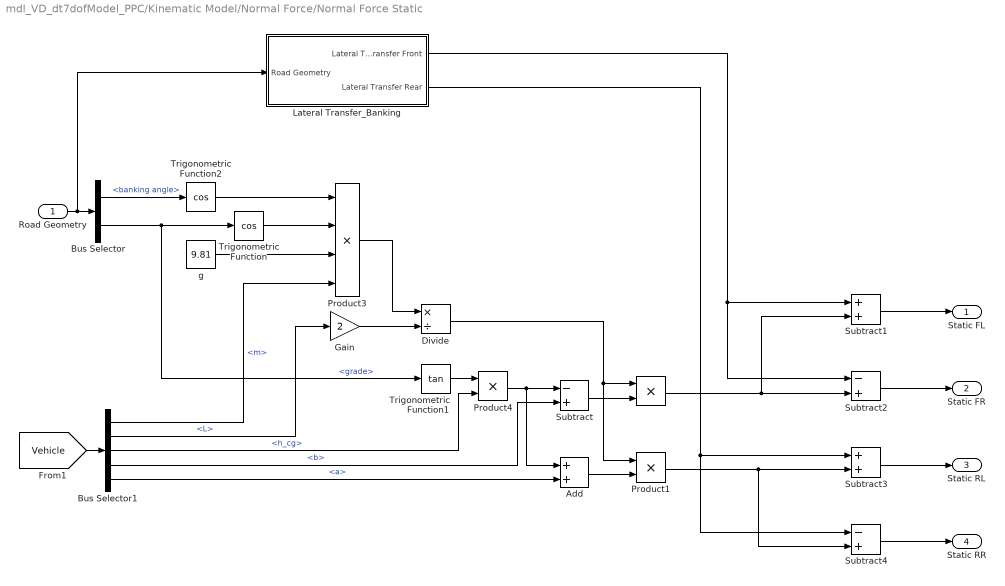
== system mdl_VD_dt7dofModel_PPC/Kinematic Model/Normal Force/Normal Force Static ==
  Road Geometry : Inport
  " " : Product  RndMeth=Zero
  Add : Sum
  Bus Selector : BusSelector  OutputSignals=road geometry.banking angle,road geometry.grade
  Bus Selector1 : BusSelector  OutputSignals=m,L,h_cg,b,a
  Divide : Product  Inputs=*/
  Gain : Gain  Gain=2
  Lateral Transfer_Banking : Subsystem
  Product1 : Product  RndMeth=Zero
  Product3 : Product  Inputs=4  RndMeth=Zero
  Product4 : Product  RndMeth=Zero
  Subtract : Sum  Inputs=-+
  Subtract1 : Sum
  Subtract2 : Sum  Inputs=-+
  Subtract3 : Sum
  Subtract4 : Sum  Inputs=-+
  Trigonometric Function : Trigonometry  Operator=cos
  Trigonometric Function1 : Trigonometry  Operator=tan
  Trigonometric Function2 : Trigonometry  Operator=cos
  g : Constant  Value=9.81
  Static FL : Outport
  Static FR : Outport  Port=2
  Static RL : Outport  Port=3
  Static RR : Outport  Port=4
  wires:
  Product4/1 -> Add/1, Subtract/1
  Add/1 -> Product1/2
  g/1 -> Product3/3
  [Vehicle] -> Bus Selector1/1
  Bus Selector1/4 -> Subtract/2  "<b>"
  Product3/1 -> Divide/1
  Bus Selector1/1 -> Product3/4  "<m>"
  Trigonometric Function/1 -> Product3/2
  Bus Selector1/5 -> Add/2  "<a>"
  Bus Selector1/3 -> Product4/2  "<h_cg>"
  Trigonometric Function1/1 -> Product4/1
  Divide/1 -> Product1/1, " "/1
  Bus Selector/2 -> Trigonometric Function1/1, Trigonometric Function/1  "<grade>"
  Bus Selector1/2 -> Gain/1  "<L>"
  Subtract/1 -> " "/2
  Gain/1 -> Divide/2
  Road Geometry/1 -> Lateral Transfer_Banking/1(Road Geometry), Bus Selector/1
  Product1/1 -> Subtract4/2, Subtract3/2
  " "/1 -> Subtract2/2, Subtract1/2
  Trigonometric Function2/1 -> Product3/1
  Bus Selector/1 -> Trigonometric Function2/1  "<banking angle>"
  Subtract4/1 -> Static RR/1
  Subtract3/1 -> Static RL/1
  Subtract2/1 -> Static FR/1
  Subtract1/1 -> Static FL/1
  Lateral Transfer_Banking/2(Lateral Transfer Rear) -> Subtract3/1, Subtract4/1
  Lateral Transfer_Banking/1(Lateral Transfer Front) -> Subtract2/1, Subtract1/1

== system mdl_VD_dt7dofModel_PPC/Kinematic Model/Vehicle Body Newtonian Dynamics/4 Wheel ax ==
  "Fx " : Inport
  Road Grade : Inport  Port=2
  Bank Angle : Inport  Port=3
  Add2 : Sum  Inputs=-+
  Bus Selector6 : BusSelector  OutputSignals=m
  Bus Selector7 : BusSelector  OutputSignals=m
  Divide2 : Product  Inputs=/*
  Product10 : Product  Inputs=4  RndMeth=Zero
  Sum of Elements3 : Sum  Inputs=+
  cos : Trigonometry  Operator=cos
  g : Constant  Value=9.81
  sin : Trigonometry
  ax : Outport
  wires:
  [Vehicle] -> Bus Selector6/1
  [Vehicle] -> Bus Selector7/1
  Add2/1 -> Divide2/2
  Bus Selector7/1 -> Divide2/1  "<m>"
  Divide2/1 -> ax/1
  Product10/1 -> Add2/1
  Sum of Elements3/1 -> Add2/2
  Bus Selector6/1 -> Product10/4  "<m>"
  g/1 -> Product10/3
  sin/1 -> Product10/1
  cos/1 -> Product10/2
  Bank Angle/1 -> cos/1
  Road Grade/1 -> sin/1
  "Fx "/1 -> Sum of Elements3/1

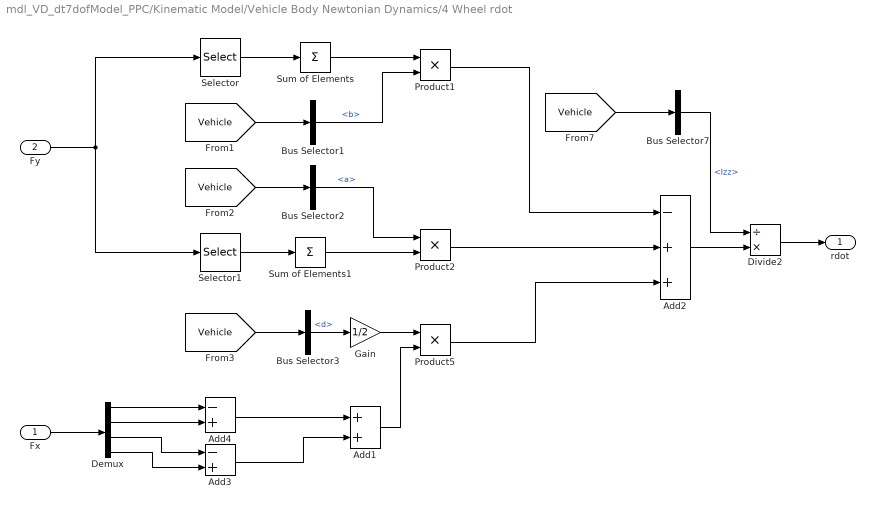
== system mdl_VD_dt7dofModel_PPC/Kinematic Model/Vehicle Body Newtonian Dynamics/4 Wheel rdot ==
  Fx : Inport
  Fy : Inport  Port=2
  Add1 : Sum
  Add2 : Sum  Inputs=-++
  Add3 : Sum  Inputs=-+
  Add4 : Sum  Inputs=-+
  Bus Selector1 : BusSelector  OutputSignals=b
  Bus Selector2 : BusSelector  OutputSignals=a
  Bus Selector3 : BusSelector  OutputSignals=d
  Bus Selector7 : BusSelector  OutputSignals=Izz
  Demux : Demux
  Divide2 : Product  Inputs=/*
  Gain : Gain  Gain=1/2
  Product1 : Product  RndMeth=Zero
  Product2 : Product  RndMeth=Zero
  Product5 : Product  RndMeth=Zero
  Selector : Selector  InputPortWidth=4  IndexOptions=Index vector (dialog)  Indices=[3 4]  OutputSizes=1
  Selector1 : Selector  InputPortWidth=4  IndexOptions=Index vector (dialog)  Indices=[1 2]  OutputSizes=1
  Sum of Elements : Sum  Inputs=+
  Sum of Elements1 : Sum  Inputs=+
  rdot : Outport
  wires:
  Fy/1 -> Selector/1, Selector1/1
  Divide2/1 -> rdot/1
  Bus Selector7/1 -> Divide2/1  "<Izz>"
  Add2/1 -> Divide2/2
  [Vehicle] -> Bus Selector7/1
  [Vehicle] -> Bus Selector1/1
  Selector/1 -> Sum of Elements/1
  Selector1/1 -> Sum of Elements1/1
  Sum of Elements/1 -> Product1/1
  Bus Selector1/1 -> Product1/2  "<b>"
  Product1/1 -> Add2/1
  Fx/1 -> Demux/1
  [Vehicle] -> Bus Selector2/1
  Product2/1 -> Add2/2
  Bus Selector2/1 -> Product2/1  "<a>"
  Sum of Elements1/1 -> Product2/2
  Demux/3 -> Add3/1
  Demux/4 -> Add3/2
  Demux/1 -> Add4/1
  Demux/2 -> Add4/2
  Add4/1 -> Add1/1
  [Vehicle] -> Bus Selector3/1
  Add1/1 -> Product5/2
  Bus Selector3/1 -> Gain/1  "<d>"
  Gain/1 -> Product5/1
  Product5/1 -> Add2/3
  Add3/1 -> Add1/2

== system mdl_VD_dt7dofModel_PPC/ST Trajectory Query/ST Trajectory Query1/Vehicle Parameters ==
  In1 : Inport
  Bus Creator1 : BusCreator  Inputs=11
  Bus Selector : BusSelector  OutputSignals=L,d
  Constant : Constant  Value=vehicle.m
  Constant1 : Constant  Value=vehicle.Izz
  Constant13 : Constant  Value=vehicle.Re
  Constant14 : Constant  Value=vehicle.h_cg
  Constant2 : Constant  Value=0.6
  Constant3 : Constant  Value=0.4
  Constant7 : Constant  Value=vehicle.Ca
  Constant8 : Constant  Value=vehicle.Cx
  Constant9 : Constant  Value=vehicle.Iw
  Product : Product
  Product1 : Product
  Vehicle : Outport
  wires:
  Bus Creator1/1 -> Vehicle/1
  Constant/1 -> Bus Creator1/1  "m"
  Constant1/1 -> Bus Creator1/2  "Izz"
  Constant9/1 -> Bus Creator1/3  "Iw"
  Constant13/1 -> Bus Creator1/4  "Re"
  Bus Selector/1 -> Product/2, Product1/1, Bus Creator1/6  "<L>"
  Constant14/1 -> Bus Creator1/9  "h_cg"
  Constant7/1 -> Bus Creator1/10  "Ca"
  Constant8/1 -> Bus Creator1/11  "Cx"
  Product/1 -> Bus Creator1/5  "a"
  Bus Selector/2 -> Bus Creator1/8  "<d>"
  Product1/1 -> Bus Creator1/7  "b"
  In1/1 -> Bus Selector/1
  Constant2/1 -> Product1/2
  Constant3/1 -> Product/1

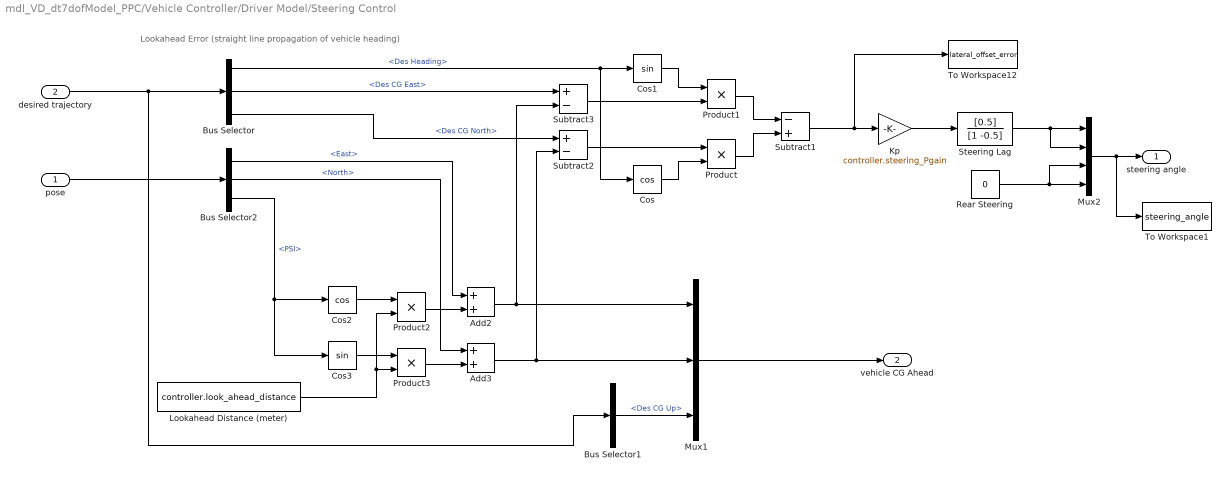
== system mdl_VD_dt7dofModel_PPC/Vehicle Controller/Driver Model/Steering Control ==
  note: Lookahead Error (straight line propagation of vehicle heading)
  pose : Inport
  desired trajectory : Inport  Port=2
  Add2 : Sum
  Add3 : Sum
  Bus Selector : BusSelector  OutputSignals=Des Heading,Des CG East,Des CG North
  Bus Selector1 : BusSelector  OutputSignals=Des CG Up
  Bus Selector2 : BusSelector  OutputSignals=East,North,PSI
  Cos : Trigonometry  Operator=cos
  Cos1 : Trigonometry
  Cos2 : Trigonometry  Operator=cos
  Cos3 : Trigonometry
  Kp : Gain  Gain=controller.steering_Pgain
  Lookahead Distance (meter) : Constant  Value=controller.look_ahead_distance
  Mux1 : Mux  Inputs=3
  Mux2 : Mux
  Product{,1..3} (4 alike) : Product
  Rear Steering : Constant  Value=0
  Steering Lag : DiscreteFilter  Numerator=[0.5]  Denominator=[1 -0.5]
  Subtract1 : Sum  Inputs=-+
  Subtract2 : Sum  Inputs=+-
  Subtract3 : Sum  Inputs=+-
  To Workspace1 : ToWorkspace  VariableName=steering_angle  SampleTime=-1
      settings: Save2DSignal=2-D array (concatenate along first dimension)
  To Workspace12 : ToWorkspace  VariableName=lateral_offset_error  SampleTime=-1
      settings: Save2DSignal=2-D array (concatenate along first dimension)
  steering angle : Outport
  vehicle CG Ahead : Outport  Port=2
  wires:
  Kp/1 -> Steering Lag/1
  Subtract2/1 -> Product/1
  Mux2/1 -> To Workspace1/1, steering angle/1
  Lookahead Distance (meter)/1 -> Product2/2, Product3/2
  Bus Selector/2 -> Subtract3/1  "<Des CG East>"
  Subtract3/1 -> Product1/2
  Cos1/1 -> Product1/1
  Add3/1 -> Subtract2/2, Mux1/2
  Bus Selector2/1 -> Add2/1  "<East>"
  Add2/1 -> Subtract3/2, Mux1/1
  Bus Selector2/2 -> Add3/1  "<North>"
  Cos3/1 -> Product3/1
  Rear Steering/1 -> Mux2/3, Mux2/4
  desired trajectory/1 -> Bus Selector/1, Bus Selector1/1
  Product/1 -> Subtract1/2
  Bus Selector2/3 -> Cos3/1, Cos2/1  "<PSI>"
  pose/1 -> Bus Selector2/1
  Cos2/1 -> Product2/1
  Product3/1 -> Add3/2
  Subtract1/1 -> To Workspace12/1, Kp/1
  Product2/1 -> Add2/2
  Product1/1 -> Subtract1/1
  Bus Selector/3 -> Subtract2/1  "<Des CG North>"
  Bus Selector/1 -> Cos/1, Cos1/1  "<Des Heading>"
  Cos/1 -> Product/2
  Steering Lag/1 -> Mux2/1, Mux2/2
  Mux1/1 -> vehicle CG Ahead/1
  Bus Selector1/1 -> Mux1/3  "<Des CG Up>"

== system mdl_VD_dt7dofModel_PPC/Vehicle Controller/Driver Model/Velocity Control ==
  desired velocity : Inport
  speeds : Inport  Port=2
  Bus Selector1 : BusSelector  OutputSignals=Des Velocity
  Bus Selector2 : BusSelector  OutputSignals=speeds.Vx
  Front Wheel Torque : Constant  Value=0
  Gain : Gain  Gain=controller.velocity_Pgain
  Mux2 : Mux
  Subtract1 : Sum  Inputs=+-
  wheel torque : Outport
  wires:
  Mux2/1 -> wheel torque/1
  Gain/1 -> Mux2/3, Mux2/4
  Subtract1/1 -> Gain/1
  desired velocity/1 -> Bus Selector1/1
  Front Wheel Torque/1 -> Mux2/2, Mux2/1
  Bus Selector1/1 -> Subtract1/1  "<Des Velocity>"
  Bus Selector2/1 -> Subtract1/2  "<Vx>"
  speeds/1 -> Bus Selector2/1
